simulink model "LPVMPC_AGV_simulink_ref"  (R2024b)
settings: Solver=ode4  StartTime=0.0  StopTime=150  FixedStep=0.01  RelTol=1e-3
PreLoadFcn:
  | preloadfcn_v2
model workspace (MAT data in the model file):
  CdA = 0.5
  MPC_idx = [1 2 3 4]
  c_r = 0.015
  db_rt.A = [1 1 1 1 1 1 1 1 1 1 1 1 ... (2000 elements, 5x5x5x4x4)]
  db_rt.B = [1.10696819051e-09 6.56859347141e-11 7.70788358052e-11 4.63456222969e-11 -1.91478442817e-11 3.08062125377e-10 3.17967815903e-10 3.27251111689e-10 3.36091973111e-10 3.44604983367e-10 -2.40695313568e-13 -1.34215112609e-13 ... (1000 elements, 5x5x5x4x2)]
  db_rt.C = [1 1 1 1 1 1 1 1 1 1 1 1 ... (2000 elements, 5x5x5x4x4)]
  db_rt.D = [0 0 0 0 0 0 0 0 0 0 0 0 ... (1000 elements, 5x5x5x4x2)]
  db_rt.E = [2.11033585519e-07 -6.42122832244e-08 -7.53495772598e-08 -4.53058513965e-08 1.871832239e-08 -3.01151562194e-07 -3.10835010863e-07 -3.19910021986e-07 -3.2855251907e-07 -3.36874515032e-07 2.35296065713e-10 1.31204413144e-10 ... (500 elements, 5x5x5x4)]
  db_rt.grid.V = [0.8; 0.9; 1; 1.1; 1.2]
  db_rt.grid.W = [-0.2; -0.1; 0; 0.1; 0.2]
  db_rt.grid.T = [-0.1; -0.05; 0; 0.05; 0.1]
  db_rt.Ts = 0.01
  db_rt.nx = 4
  db_rt.nu = 2
  db_rt.ny = 4
  db_rt.nd = 1
  db_rt.Nv = 5
  db_rt.Nw = 5
  db_rt.Nt = 5
  g = 9.81
  m = 100
  rho = 1.225
undefined symbols (not defined in the file): ff_rt, params, v_ff_nom
libraries: mpclib x1
settings Model: Creator=15754  LastModifiedBy=15754

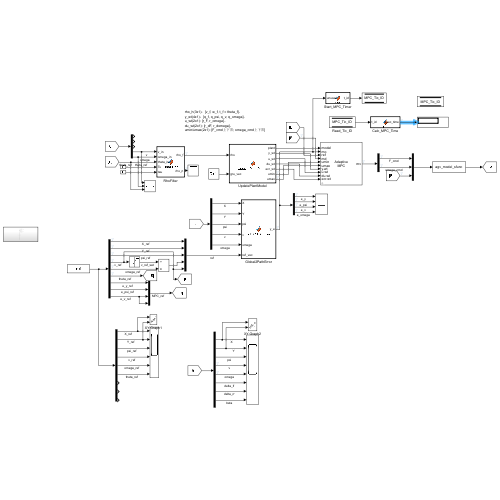
[thumbnail: Simulink's stored preview of the top-level diagram]
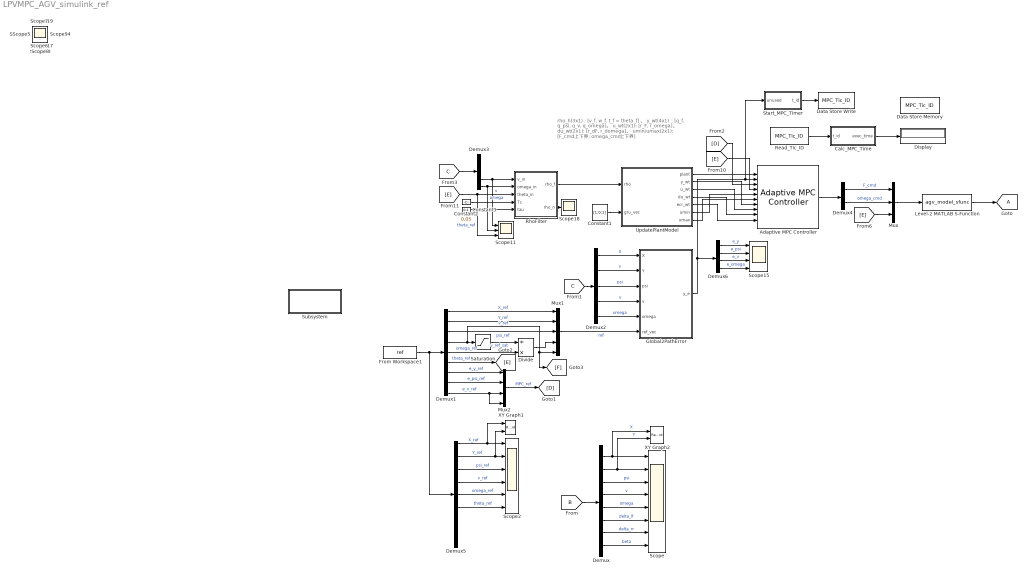
== system LPVMPC_AGV_simulink_ref ==
  note: rho_h(3x1)：[v_f, w_f, t_f = theta_f]。
      | y_wt(4x1)：[q_f, q_psi, q_v, q_omega]。
      | u_wt(2x1): [r_F, r_omega]。
      | du_wt(2x1): [r_dF, r_domega]。
      | umin/umax(2x1): [F_cmd上下界; omega_cmd上下界]
  Adaptive MPC Controller : mpclib/Adaptive MPC Controller  SCDEnableBlockLinearizationSpecification=on  mpcobj=ctrl.mpcobj  enable_value=0  updateMPCinCallerWorkspace=on  md_inport=on  mv_inport=off  uref_inport=off  return_cost=off  return_mvseq=off  return_qpstatus=off  return_xseq=off  return_state=off  return_ovseq=off  state_inport=off  isltv_plant=off  umin_inport=on  umax_inport=on  ymin_inport=off  ymax_inport=off  cc_inport=off  ywt_inport=on  uwt_inport=on  duwt_inport=on  rhoeps_inport=on  pm_inport=off  MaximumP=10  HorizonChoice=FixedHorizon  BlockDataType=double  SampleTimeInherited=off  switch_inport=off
  Calc_MPC_Time : MATLAB Function  TreatAsAtomicUnit=on
  Constant1 : Constant  Value=[1;0;1]
  Constant2 : Constant  Value=0.05  SampleTime=params.Ts
  Constant3 : Constant  Value=0.4  SampleTime=params.Ts
  Data Store Memory : DataStoreMemory  DataStoreName=MPC_Tic_ID  WriteAfterWriteMsg=warning  ShowAdditionalParam=off  OutDataTypeStr=uint64  DataLoggingName=solve_time_ms
      settings: DataLoggingNameMode=Custom
  Data Store Write : DataStoreWrite  DataStoreName=MPC_Tic_ID  IndexOptions=Index vector (dialog)  Indices=1  OutputSizes=1
  Demux : Demux  Outputs=8
  Demux1 : Demux  Outputs=9
  Demux2 : Demux  Outputs=5
  Demux3 : Demux  Outputs=5
  Demux4 : Demux  Outputs=2
  Demux5 : Demux  Outputs=9
  Demux6 : Demux
  Display : Display
  Divide : Product  Inputs=/*
  From Workspace1 : FromWorkspace  VariableName=ref  SampleTime=0.05
  Global2PathError : MATLAB Function  TreatAsAtomicUnit=on  SystemSampleTime=params.Ts
  Goto : Goto  TagVisibility=global
  Level-2 MATLAB S-Function : M-S-Function  FunctionName=agv_model_sfunc  Parameters=parameters
  Mux : Mux  Inputs=3
  Mux1 : Mux  Inputs=5
  Mux2 : Mux
  Read_Tic_ID : DataStoreRead  DataStoreName=MPC_Tic_ID  IndexOptions=Index vector (dialog)  Indices=1  OutputSizes=1
  RhoFilter : MATLAB Function  TreatAsAtomicUnit=on  SystemSampleTime=0.05
  Saturation : Saturate  UpperLimit=Inf  LowerLimit=1e-3
  Scope : Scope  NumInputPorts=8
  Scope11 : Scope  NumInputPorts=3
  Scope15 : Scope  NumInputPorts=4
  Scope{1,3..9,12..14,16..19} (15 alike) : Scope
  Scope2 : Scope  NumInputPorts=6
  Start_MPC_Timer : MATLAB Function  TreatAsAtomicUnit=on
  Subsystem : Subsystem
  UpdatePlantModel : MATLAB Function  TreatAsAtomicUnit=on
  XY Graph1 : Record  FileSettingsInternal="{\"entries\":[{\"content\":{\"excelSettings\":{\"content\":{},\"type\":\"Streamout.ExcelSettings\"}},\"type\":\"Streamout.FileSettingStorage\",\"uuid\":\"\"}],\"packageUris\":[\"http:\\/\\/schema.mathworks.com\\/mf0\\/streamout_blocks\\/R2020a\"],\"version\":\"1.0\"}"  Layout=[1 1]  SignalsInternal="{\"entries\":[{\"content\":{\"signals\":[{\"content\":{\"blockPath\":[],\"dimensions\":[1],\"domain\":\"\",\"lineColor\":\"#a2142f\",\"plots\":[ 1 ],\"port\":1,\"signalID\":1,\"signalName\":\"X_ref\"},\"type\":\"RecordBlkView.Signal\",\"uuid\":\"\"},{\"content\":{\"blockPath\":[],\"dimensions\":[1],\"domain\":\"\",\"lineColor\":\"#139fff\",\"plots\":[ 1 ],\"port\":2,\"signalID\":2,\"signalName\":\"Y_ref\"},\"type\":\"RecordBlkView.Signal\",\"uuid\":\"\"}]},\"type\":\"RecordBlkView.InputSignals\",\"uuid\":\"\"}],\"packageUris\":[\"http:\\/\\/schema.mathworks.com\\/mf0\\/streamout_blocks\\/R2020a\"],\"version\":\"1.0\"}"  VisualizationBindings="{\"xyplotplugin\":{\"info\":[{\"series\":[{\"bindingParametersList\":[{\"parameter\":\"X-Axis\",\"signalID\":1,\"signalName\":\"X_ref\"},{\"parameter\":\"Y-Axis\",\"signalID\":2,\"signalName\":\"Y_ref\"}],\"seriesID\":0}],\"subplotID\":1}]}}"  CompatibilityTag=XY
  XY Graph2 : Record  FileSettingsInternal="{\"entries\":[{\"content\":{\"excelSettings\":{\"content\":{},\"type\":\"Streamout.ExcelSettings\"}},\"type\":\"Streamout.FileSettingStorage\",\"uuid\":\"\"}],\"packageUris\":[\"http:\\/\\/schema.mathworks.com\\/mf0\\/streamout_blocks\\/R2020a\"],\"version\":\"1.0\"}"  Layout=[1 1]  SignalsInternal="{\"entries\":[{\"content\":{\"signals\":[{\"content\":{\"blockPath\":[],\"dimensions\":[1],\"domain\":\"\",\"lineColor\":\"#a2142f\",\"plots\":[ 1 ],\"port\":1,\"signalID\":1,\"signalName\":\"X\"},\"type\":\"RecordBlkView.Signal\",\"uuid\":\"\"},{\"content\":{\"blockPath\":[],\"dimensions\":[1],\"domain\":\"\",\"lineColor\":\"#139fff\",\"plots\":[ 1 ],\"port\":2,\"signalID\":2,\"signalName\":\"Y\"},\"type\":\"RecordBlkView.Signal\",\"uuid\":\"\"}]},\"type\":\"RecordBlkView.InputSignals\",\"uuid\":\"\"}],\"packageUris\":[\"http:\\/\\/schema.mathworks.com\\/mf0\\/streamout_blocks\\/R2020a\"],\"version\":\"1.0\"}"  VisualizationBindings="{\"xyplotplugin\":{\"info\":[{\"series\":[{\"bindingParametersList\":[{\"parameter\":\"X-Axis\",\"signalID\":1,\"signalName\":\"X\"},{\"parameter\":\"Y-Axis\",\"signalID\":2,\"signalName\":\"Y\"}],\"seriesID\":0}],\"subplotID\":1}]}}"  CompatibilityTag=XY
  wires:
  UpdatePlantModel/1(plant) -> Adaptive MPC Controller/1
  UpdatePlantModel/7(umax) -> Adaptive MPC Controller/6
  Demux2/5 -> Global2PathError/5(omega)  "omega"
  Demux/8 -> Scope/8  "beta"
  [E] -> Mux/3
  UpdatePlantModel/5(ecr_wt) -> Adaptive MPC Controller/10
  Demux/3 -> Scope/3  "psi"
  Mux2/1 -> [D]  "MPC_ref"
  Demux4/2 -> Mux/2  "omega_cmd"
  Level-2 MATLAB S-Function/1 -> Goto/1
  Demux6/1 -> Scope15/1  "e_y"
  Demux1/5 -> Divide/2  "omega_ref"
  RhoFilter/1(rho_f) -> UpdatePlantModel/1(rho)
  Demux6/3 -> Scope15/3  "e_v"
  Demux5/4 -> Scope2/4  "v_ref"
  Demux/5 -> Scope/5  "omega"
  Demux5/5 -> Scope2/5  "omega_ref"
  Demux2/4 -> Global2PathError/4(v)  "v"
  Demux5/1 -> XY Graph1/1, Scope2/1  "X_ref"
  UpdatePlantModel/4(du_wt) -> Adaptive MPC Controller/9
  Demux3/5 -> Scope11/2, RhoFilter/2(omega_in)  "omega"
  Constant2/1 -> RhoFilter/4(Ts)
  Demux1/7 -> Mux2/1  "e_y_ref"
  Demux1/3 -> Mux1/3  "psi_ref"
  Demux3/4 -> Scope11/1, RhoFilter/1(v_in)  "v"
  Adaptive MPC Controller/1 -> Demux4/1
  Demux/7 -> Scope/7  "delta_rr"
  Mux1/1 -> Global2PathError/6(ref_vec)  "ref"
  Demux2/2 -> Global2PathError/2(Y)  "Y"
  [B] -> Demux/1
  Constant1/1 -> UpdatePlantModel/2(gru_vec)
  [E] -> Scope11/3, RhoFilter/3(theta_in)  "theta_ref"
  Demux/1 -> XY Graph2/1, Scope/1  "X"
  Demux1/8 -> Mux2/2  "e_psi_ref"
  Demux5/2 -> XY Graph1/2, Scope2/2  "Y_ref"
  Demux2/3 -> Global2PathError/3(psi)  "psi"
  From Workspace1/1 -> Demux5/1, Demux1/1
  Demux6/2 -> Scope15/2  "e_psi"
  Demux5/3 -> Scope2/3  "psi_ref"
  Saturation/1 -> Divide/1  "v_ref_sat"
  Demux/6 -> Scope/6  "delta_lf"
  Demux1/6 -> [E]  "theta_ref"
  UpdatePlantModel/2(y_wt) -> Adaptive MPC Controller/7
  Demux1/9 -> Mux2/4, Mux2/3  "e_v_ref"
  Demux5/6 -> Scope2/6  "theta_ref"
  Demux1/2 -> Mux1/2  "Y_ref"
  [C] -> Demux3/1
  Demux2/1 -> Global2PathError/1(X)  "X"
  Divide/1 -> Mux1/4
  UpdatePlantModel/3(u_wt) -> Adaptive MPC Controller/8
  Demux6/4 -> Scope15/4  "e_omega"
  Demux/4 -> Scope/4  "v"
  Constant3/1 -> RhoFilter/5(tau)
  [C] -> Demux2/1
  [D] -> Adaptive MPC Controller/3
  Demux4/1 -> Mux/1  "F_cmd"
  UpdatePlantModel/6(umin) -> Adaptive MPC Controller/5
  Demux1/1 -> Mux1/1  "X_ref"
  RhoFilter/2(rho_n) -> Scope18/1
  Demux/2 -> XY Graph2/2, Scope/2  "Y"
  Demux1/4 -> [F], Mux1/5, Saturation/1  "v_ref"
  Mux/1 -> Level-2 MATLAB S-Function/1
  [E] -> Adaptive MPC Controller/4
  Read_Tic_ID/1 -> Calc_MPC_Time/1(t_id)
  Calc_MPC_Time/1(exec_time) -> Display/1
  Global2PathError/1(y_e) -> Demux6/1, Start_MPC_Timer/1(unused), Adaptive MPC Controller/2
  Start_MPC_Timer/1(t_id) -> Data Store Write/1

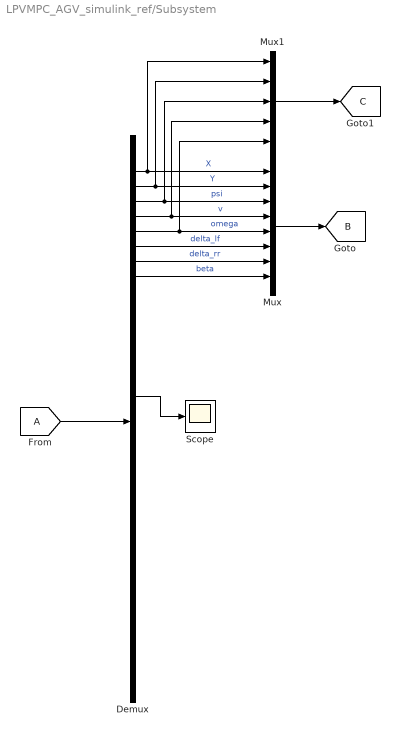
== system LPVMPC_AGV_simulink_ref/Subsystem ==
  Demux : Demux  Outputs=34
  From : From  TagVisibility=global
  Mux : Mux  Inputs=8
  Mux1 : Mux  Inputs=5
  Scope : Scope
  tag scope: B=global, C=global
  wires:
  From/1 -> Demux/1
  Demux/1 -> Mux/1, Mux1/1  "X"
  Demux/2 -> Mux/2, Mux1/2  "Y"
  Demux/3 -> Mux/3, Mux1/3  "psi"
  Demux/4 -> Mux/4, Mux1/4  "v"
  Demux/5 -> Mux/5, Mux1/5  "omega"
  Demux/6 -> Mux/6  "delta_lf"
  Demux/7 -> Mux/7  "delta_rr"
  Demux/8 -> Mux/8  "beta"
  Mux/1 -> [B]
  Mux1/1 -> [C]
  Demux/16 -> Scope/1

== matlab function LPVMPC_AGV_simulink_ref/RhoFilter ==
  data: v_in input; rho_f output; omega_in input; theta_in input; Ts input; tau input; rho_n output
function [rho_f, rho_n] = RhoFilter(v_in, omega_in, theta_in, Ts, tau)
% 一阶离散滤波
persistent v_f_prev w_f_prev t_f_prev
if isempty(v_f_prev), v_f_prev = 0; end
if isempty(w_f_prev), w_f_prev = 0; end
if isempty(t_f_prev), t_f_prev = 0; end

a = Ts / max(tau + Ts, 1e-6);

v_f = (1 - a)*v_f_prev + a*max(v_in, 0);   % 速度不取负·
w_f = (1 - a)*w_f_prev + a*omega_in;       % 保留符号
t_f = (1 - a)*t_f_prev + a*theta_in;       % 保留符号

v_f_prev = v_f; w_f_prev = w_f; t_f_prev = t_f;

rho_f = [v_f; w_f; t_f];

% 可选归一化（仅用于监控/调试，不参与UpdatePlantModel）
Vmax = 2.0; Wmax = 0.8; Tmax = deg2rad(10);
rho_n = [min(v_f/Vmax,1); min(abs(w_f)/Wmax,1); min(abs(t_f)/Tmax,1)];
end

== matlab function LPVMPC_AGV_simulink_ref/Global2PathError ==
  data: X input; y_e output; Y input; psi input; v input; omega input; ref_vec input
% 误差计算模块
function y_e = Global2PathError(X, Y, psi, v, omega, ref_vec)
% ref_vec = [X_ref; Y_ref; psi_ref; kappa_ref; v_ref]
% 输出: y_e = [e_y; e_psi; e_v; e_omega; e_s]

%#codegen
% 1) 解包参考
Xr = ref_vec(1);
Yr = ref_vec(2);
psir = ref_vec(3);
kappa = ref_vec(4);
v_ref = ref_vec(5);

% 2) 横向误差：沿参考法向量投影（带符号）
ex = X - Xr; 
ey = Y - Yr;
e_y = -sin(psir)*ex + cos(psir)*ey;

% 3) 航向、速度、角速度误差
e_psi   = wrapToPi(psi - psir);
e_v     = v - v_ref;
omega_ff= v_ref * kappa;           % 曲率前馈
e_omega = omega - omega_ff;

% 4) 进度误差（可选，如未使用可置 0）
e_s = 0;

y_e = [e_y; e_psi; e_v; e_omega];
end

== matlab function LPVMPC_AGV_simulink_ref/UpdatePlantModel ==
  data: rho input; gru_vec input; plant output Bus: MPCPlantBus; db_rt parameter; MPC_idx parameter double size=[1 4]; ff_rt parameter; v_ff_nom parameter; y_wt output; u_wt output; du_wt output; ecr_wt output; umin output; umax output
function [plant, y_wt, u_wt, du_wt, ecr_wt, umin, umax] = UpdatePlantModel(rho, gru_vec, db_rt, MPC_idx, ff_rt, v_ff_nom)
%#codegen
% gru_vec = [label_main; label_turn; conf_main]

gv = [1; 0; 1]; % 默认: flat / straight / high confidence
if ~isempty(gru_vec)
g = double(gru_vec(:));
n = min(3, numel(g));
gv(1:n) = g(1:n);
end

[plant, y_wt, u_wt, du_wt, ecr_wt, umin, umax] = UpdatePlantModel_gru( ...
rho, db_rt, MPC_idx, ff_rt, v_ff_nom, gv);
end

== matlab function LPVMPC_AGV_simulink_ref/Start_MPC_Timer ==
  data: unused input; t_id output
function t_id = fcn(~)
%#codegen
% 声明tic为 extrinsic 函数，避免代码生成报错
coder.extrinsic('tic');
t_id = uint64(0);
t_id = tic; % 启动计时器，获取句柄

== matlab function LPVMPC_AGV_simulink_ref/Calc_MPC_Time ==
  data: t_id input; exec_time output
function exec_time = fcn(t_id)
%#codegen
% 声明toc为 extrinsic 函数
coder.extrinsic('toc');
exec_time = 0;
exec_time = toc(t_id); % 计算耗时，单位：秒
